simulink model "LSTM_import_smc"  (R2022a)
settings: Solver=VariableStepAuto  StartTime=0.0  StopTime=100  RelTol=1e-3
values from neighbouring files (symbols this model uses):
  Temp_lstm = lstmLayer(numHidden,"CellState",zeros(numHidden,1),"HiddenState",zeros(numHidden,1))    [LSTM_import.m]    (also in LSTM_import_layer2.m)
libraries: deeplib x1
settings Model: Creator=User  LastModifiedBy=User

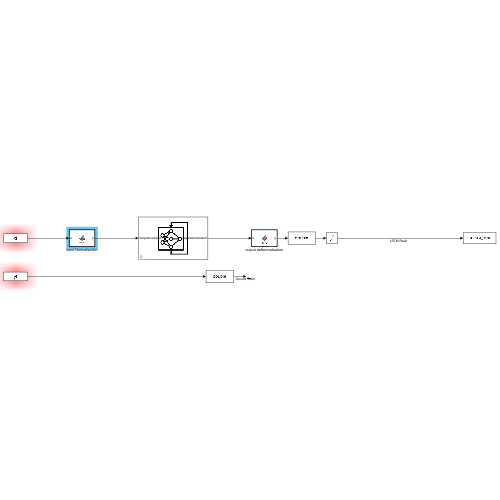
[thumbnail: Simulink's stored preview of the top-level diagram]
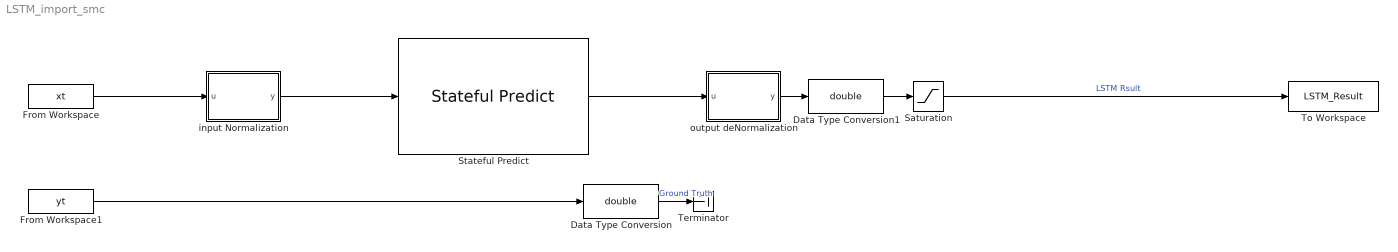
== system LSTM_import_smc ==
  Data Type Conversion : DataTypeConversion  OutDataTypeStr=double  SaturateOnIntegerOverflow=off  RndMeth=Floor
  Data Type Conversion1 : DataTypeConversion  OutDataTypeStr=double  SaturateOnIntegerOverflow=off  RndMeth=Floor
  From Workspace : FromWorkspace  VariableName=xt  SampleTime=0.1
  From Workspace1 : FromWorkspace  VariableName=yt  SampleTime=0.1
  Saturation : Saturate  UpperLimit=2400  LowerLimit=-2400
  Stateful Predict : deeplib/Stateful Predict  Network=Network from MAT-file  NetworkFunction=untitled  NetworkFilePath=C:\Users\User\Desktop\Code\TV\CARMAKER\Temp_lstm.mat  InputDataFormats={ '', '' }  SampleTime=0.1  ForceInterpretedSim=off  EnableDLNetwork=on
      settings: SourceProductBaseCode=NN
  Terminator : Terminator
  To Workspace : ToWorkspace  VariableName=LSTM_Result  SaveFormat=Timeseries  SampleTime=-1
  input Normalization : MATLAB Function  TreatAsAtomicUnit=on
  output deNormalization : MATLAB Function  TreatAsAtomicUnit=on
  wires:
  From Workspace/1 -> input Normalization/1(u)
  input Normalization/1(y) -> Stateful Predict/1
  Saturation/1 -> To Workspace/1  "LSTM Rsult"
  From Workspace1/1 -> Data Type Conversion/1
  Stateful Predict/1 -> output deNormalization/1(u)
  output deNormalization/1(y) -> Data Type Conversion1/1
  Data Type Conversion1/1 -> Saturation/1
  Data Type Conversion/1 -> Terminator/1  "Ground Truth"

== matlab function LSTM_import_smc/output deNormalization ==
  data: u input; y output
function y = fcn(u)

x_min = double(-2400);  
x_max = double(2400);

y = x_min + (x_max-x_min).*u;

== matlab function LSTM_import_smc/input Normalization ==
  data: u input; y output
function y = fcn(u)

x_min =  [-0.53; 0; 0; 0; 0; -30; -0.26; -1.6; 0];  
x_max = [0.53; 30; 30; 30; 30; 30; 0.26; 1.6; 35];

y = (u-x_min)./(x_max-x_min);
